simulink model "HANcoder_E407_TTA_Template_group2"  (R2018b)
settings: Solver=FixedStepDiscrete  StartTime=0.0  StopTime=1  FixedStep=0.01  RelTol=1e-3
PreLoadFcn:
  | librarySetup
  | eval([bdroot,'_startup']) %Calling [modelName]_startup.m
values from neighbouring files (symbols this model uses):
  basic_cycle_duration_bc0 = TM_Reset_Board   + COMP_duration    (= 1050)    [HANcoder_E407_TTA_Group2_startup.m]    (also in HANcoder_E407_TTA_Template_startup.m = 212)
  basic_cycle_duration_bc1 = TM_Reset_Var_bc1 + COMP_duration    (= 1070)    [HANcoder_E407_TTA_Group2_startup.m]    (also in HANcoder_E407_TTA_Template_startup.m = 212)
  comm_delay_estimation1 = round(comm_delay_measured1*hardware_granularity/frequency_IRQ)    [HANcoder_E407_TTA_Group2_startup.m]    (also in HANcoder_E407_TTA_Template_startup.m)
  comm_delay_estimation2 = round(comm_delay_measured2*hardware_granularity/frequency_IRQ)    [HANcoder_E407_TTA_Group2_startup.m]    (also in HANcoder_E407_TTA_Template_startup.m)
  COMM_Period = 60    [HANcoder_E407_TTA_Group2_startup.m]    (also in HANcoder_E407_TTA_Template_startup.m = 40)
  COMM_Phase1 = Simulink.Parameter    [HANcoder_E407_TTA_Group2_startup.m]    (also in HANcoder_E407_TTA_Template_startup.m)
  COMM_Phase2 = Simulink.Parameter    [HANcoder_E407_TTA_Group2_startup.m]    (also in HANcoder_E407_TTA_Template_startup.m)
  COMM_Phase_init1 = Simulink.Parameter    [HANcoder_E407_TTA_Group2_startup.m]    (also in HANcoder_E407_TTA_Template_startup.m)
  COMM_Phase_init2 = Simulink.Parameter    [HANcoder_E407_TTA_Group2_startup.m]    (also in HANcoder_E407_TTA_Template_startup.m)
  COMP_duration = 50    [HANcoder_E407_TTA_Group2_startup.m]    (also in HANcoder_E407_TTA_Template_startup.m = 4)
  Controller1_Board = 1    [HANcoder_E407_TTA_Group2_startup.m]    (also in HANcoder_E407_TTA_Template_startup.m)
  Controller2_Board = 2    [HANcoder_E407_TTA_Group2_startup.m]    (also in HANcoder_E407_TTA_Template_startup.m)
  Controller3_Board = 3    [HANcoder_E407_TTA_Group2_startup.m]    (also in HANcoder_E407_TTA_Template_startup.m)
  delta_a_set = Simulink.Parameter    [HANcoder_E407_TTA_Group2_startup.m]
  delta_f_set = Simulink.Parameter    [HANcoder_E407_TTA_Group2_startup.m]
  delta_max = 1    [HANcoder_E407_TTA_Group2_startup.m]
  delta_min = -1    [HANcoder_E407_TTA_Group2_startup.m]
  delta_precision = 6    [HANcoder_E407_TTA_Group2_startup.m]
  frequency_IRQ = 100    [HANcoder_E407_TTA_Group2_startup.m]    (also in HANcoder_E407_TTA_Template_startup.m)
  HANtuneOverride = Simulink.Parameter    [HANcoder_E407_TTA_Group2_startup.m]    (also in HANcoder_E407_TTA_Template_startup.m)
  idle_time_init = basic_cycle_duration_bc0 + basic_cycle_duration_bc1    (= 2120)    [HANcoder_E407_TTA_Group2_startup.m]    (also in HANcoder_E407_TTA_Template_startup.m = 424)
  Input_Gen_Board = 5    [HANcoder_E407_TTA_Group2_startup.m]
  LA_Clock_Gr = 1    [HANcoder_E407_TTA_Group2_startup.m]    (also in HANcoder_E407_TTA_Template_startup.m)
  LA_COMM_dly = 1    [HANcoder_E407_TTA_Group2_startup.m]    (also in HANcoder_E407_TTA_Template_startup.m)
  LA_COMM_Err = 1    [HANcoder_E407_TTA_Group2_startup.m]    (also in HANcoder_E407_TTA_Template_startup.m)
  LA_E_Desync = 1    [HANcoder_E407_TTA_Group2_startup.m]    (also in HANcoder_E407_TTA_Template_startup.m)
  LA_MEX_Flag = 1    [HANcoder_E407_TTA_Group2_startup.m]    (also in HANcoder_E407_TTA_Template_startup.m)
  LA_Task_Act = 1    [HANcoder_E407_TTA_Group2_startup.m]    (also in HANcoder_E407_TTA_Template_startup.m)
  Master_Role = 1    [HANcoder_E407_TTA_Group2_startup.m]    (also in HANcoder_E407_TTA_Template_startup.m)
  matrix_rows = 2    [HANcoder_E407_TTA_Group2_startup.m]    (also in HANcoder_E407_TTA_Template_startup.m)
  max_desync = 30    [HANcoder_E407_TTA_Group2_startup.m]    (also in HANcoder_E407_TTA_Template_startup.m = 15)
  max_num_msgs_CAN1 = 2^Tx_bit_number-1    (= 7)    [HANcoder_E407_TTA_Group2_startup.m]    (also in HANcoder_E407_TTA_Template_startup.m)
  max_num_msgs_CAN2 = max_num_msgs_CAN1    (= 7)    [HANcoder_E407_TTA_Group2_startup.m]    (also in HANcoder_E407_TTA_Template_startup.m)
  min_desync = (-1)*max_desync    (= -30)    [HANcoder_E407_TTA_Group2_startup.m]    (also in HANcoder_E407_TTA_Template_startup.m = -15)
  OutControl1_ID = 23    [HANcoder_E407_TTA_Group2_startup.m]    (also in HANcoder_E407_TTA_Template_startup.m)
  OutControl2_ID = 24    [HANcoder_E407_TTA_Group2_startup.m]    (also in HANcoder_E407_TTA_Template_startup.m)
  OutEmulator_ID = 25    [HANcoder_E407_TTA_Group2_startup.m]    (also in HANcoder_E407_TTA_Template_startup.m)
  script_run = Simulink.Parameter    [HANcoder_E407_TTA_Group2_startup.m]    (also in HANcoder_E407_TTA_Template_startup.m)
  SensorValues_ID = 22    [HANcoder_E407_TTA_Group2_startup.m]    (also in HANcoder_E407_TTA_Template_startup.m)
  SetValues_ID = 21    [HANcoder_E407_TTA_Group2_startup.m]    (also in HANcoder_E407_TTA_Template_startup.m)
  Slave_Role = 3    [HANcoder_E407_TTA_Group2_startup.m]    (also in HANcoder_E407_TTA_Template_startup.m = 2)
  speed_max = 10    [HANcoder_E407_TTA_Group2_startup.m]
  speed_min = -10    [HANcoder_E407_TTA_Group2_startup.m]
  speed_precision = 3    [HANcoder_E407_TTA_Group2_startup.m]
  Sync_ID = 1    [HANcoder_E407_TTA_Group2_startup.m]    (also in HANcoder_E407_TTA_Template_startup.m)
  TM_Check_Sensor_Values = TM_COMM_Sensor_Values + COMM_duration    (= 330)    [HANcoder_E407_TTA_Group2_startup.m]
  TM_Check_Sensor_Values_2 = TM_Check_Sensor_Values + 6    (= 336)    [HANcoder_E407_TTA_Group2_startup.m]
  TM_Check_Set_Values = TM_COMM_Set_Values + COMM_duration    (= 220)    [HANcoder_E407_TTA_Group2_startup.m]
  TM_Check_Set_Values_2 = TM_Check_Set_Values + 6    (= 226)    [HANcoder_E407_TTA_Group2_startup.m]
  TM_Check_Sync = TM_COMM_Sync   + COMM_duration    (= 40)    [HANcoder_E407_TTA_Template_startup.m]
  TM_Check_TOuts = TM_Count_Vote3 + COMP_duration    (= 196)    [HANcoder_E407_TTA_Template_startup.m]
  TM_Check_Vote1 = TM_COMM_Vote1  + COMM_duration    (= 92)    [HANcoder_E407_TTA_Template_startup.m]
  TM_Check_Vote2 = TM_COMM_Vote2  + COMM_duration    (= 140)    [HANcoder_E407_TTA_Template_startup.m]
  TM_Check_Vote3 = TM_COMM_Vote3  + COMM_duration    (= 188)    [HANcoder_E407_TTA_Template_startup.m]
  TM_COMM_Set_Values = TM_bc0_3 + COMP_duration    (= 160)    [HANcoder_E407_TTA_Group2_startup.m]
  TM_COMM_Sync = basic_cycle_start    (= 0)    [HANcoder_E407_TTA_Group2_startup.m]    (also in HANcoder_E407_TTA_Template_startup.m)
  TM_COMM_Vote1 = TM_Vote_Dec    + COMP_duration    (= 52)    [HANcoder_E407_TTA_Template_startup.m]
  TM_COMM_Vote2 = TM_Count_Vote1 + COMP_duration    (= 100)    [HANcoder_E407_TTA_Template_startup.m]
  TM_COMM_Vote3 = TM_Count_Vote2 + COMP_duration    (= 148)    [HANcoder_E407_TTA_Template_startup.m]
  TM_Count_Vote1 = TM_Check_Vote1 + COMP_duration    (= 96)    [HANcoder_E407_TTA_Template_startup.m]
  TM_Count_Vote2 = TM_Check_Vote2 + COMP_duration    (= 144)    [HANcoder_E407_TTA_Template_startup.m]
  TM_Count_Vote3 = TM_Check_Vote3 + COMP_duration    (= 192)    [HANcoder_E407_TTA_Template_startup.m]
  TM_Data_bc0 = TM_COMM_Sync    (= 0)    [HANcoder_E407_TTA_Group2_startup.m]    (also in HANcoder_E407_TTA_Template_startup.m)
  TM_Data_bc1 = TM_Data_bc0(1:4)    [HANcoder_E407_TTA_Group2_startup.m]    (also in HANcoder_E407_TTA_Template_startup.m)
  TM_New_Master = TM_Check_TOuts + COMP_duration    (= 200)    [HANcoder_E407_TTA_Template_startup.m]
  TM_Reset_Board = TM_Reset_Var   + COMP_duration    (= 1000)    [HANcoder_E407_TTA_Group2_startup.m]    (also in HANcoder_E407_TTA_Template_startup.m = 208)
  TM_Reset_Var = TM_bc0_18  + COMP_duration    (= 950)    [HANcoder_E407_TTA_Group2_startup.m]    (also in HANcoder_E407_TTA_Template_startup.m = 204)
  TM_Reset_Var_bc1 = TM_bc1_19 + COMP_duration    (= 1020)    [HANcoder_E407_TTA_Group2_startup.m]    (also in HANcoder_E407_TTA_Template_startup.m = 200)
  TM_Reset_Var_bc1_2 = TM_Reset_Var_bc1 + 6    (= 1026)    [HANcoder_E407_TTA_Group2_startup.m]    (also in HANcoder_E407_TTA_Template_startup.m = 202)
  TM_Type_bc0 = COMM    (= 0)    [HANcoder_E407_TTA_Group2_startup.m]    (also in HANcoder_E407_TTA_Template_startup.m)
  TM_Type_bc1 = TM_Type_bc0(1:4)    [HANcoder_E407_TTA_Group2_startup.m]    (also in HANcoder_E407_TTA_Template_startup.m)
  TM_Update_LT = TM_Check_Sync  + COMP_duration    (= 44)    [HANcoder_E407_TTA_Template_startup.m]
  TM_Update_LT_2 = TM_Update_LT   + 2    (= 46)    [HANcoder_E407_TTA_Template_startup.m]
  TM_Vote_Dec = TM_Update_LT   + COMP_duration    (= 48)    [HANcoder_E407_TTA_Template_startup.m]
  TM_Vote_Dec_2 = TM_Vote_Dec    + 2    (= 50)    [HANcoder_E407_TTA_Template_startup.m]
  v_set = Simulink.Parameter    [HANcoder_E407_TTA_Group2_startup.m]
  Vote1_ID = 11    [HANcoder_E407_TTA_Group2_startup.m]    (also in HANcoder_E407_TTA_Template_startup.m)
  Vote2_ID = 12    [HANcoder_E407_TTA_Group2_startup.m]    (also in HANcoder_E407_TTA_Template_startup.m)
  Vote3_ID = 13    [HANcoder_E407_TTA_Group2_startup.m]    (also in HANcoder_E407_TTA_Template_startup.m)
undefined symbols (not defined in the file or in its folder): A0, A1, A2, A3, A4, CON2, CON4, D10, D12, D13, D8, D9
libraries: hdlsllib x133, HANcoder_STM32_Target x28, simulink x3, simulink_extras x1
(part 1 of 16)
CloseFcn:
  | rtwprivate ssgencode ModelCloseRequest mytest
settings Model: Creator=Jason van Kolfschoten  LastModifiedBy=moham
settings SolverCC: PositivePriorityOrder=on
settings DataIOCC: LimitDataPoints=on  SaveFormat=Array  SignalLoggingSaveFormat=ModelDataLogs  SaveOutput=off  SignalLogging=off  DSMLogging=off  SaveTime=off
settings OptimizationCC: BlockReduction=off  DefaultParameterBehavior=Inlined  DefaultUnderspecifiedDataType=single  InlineInvariantSignals=on  ExpressionDepthLimit=2147483647  StateBitsets=on  DataBitsets=on  ZeroExternalMemoryAtStartup=off  ZeroInternalMemoryAtStartup=off  InitFltsAndDblsToZero=on  NoFixptDivByZeroProtection=on  EfficientFloat2IntCast=on  LifeSpan=inf
settings DebuggingCC: SaveWithDisabledLinksMsg=none  SaveWithParameterizedLinksMsg=none  CheckSSInitialOutputMsg=off  UnderspecifiedInitializationDetection=Classic  MergeDetectMultiDrivingBlocksExec=none  SignalResolutionControl=TryResolveAll  SolverPrmCheckMsg=warning  InheritedTsInSrcMsg=none  MultiTaskDSMMsg=warning  MultiTaskCondExecSysMsg=none  ParameterPrecisionLossMsg=none  FcnCallInpInsideContextMsg=warning  BusObjectLabelMismatch=none  StateNameClashWarn=warning  SFUnexpectedBacktrackingDiag=warning  SFNoUnconditionalDefaultTransitionDiag=warning  SFExecutionAtInitializationDiag=none
settings HardwareCC: ProdBitPerPointer=32  ProdBitPerSizeT=32  ProdBitPerPtrDiffT=32  ProdLargestAtomicInteger=Long  ProdLargestAtomicFloat=Double  ProdWordSize=32  ProdHWDeviceType=ARM Compatible->ARM Cortex  TargetEndianess=LittleEndian  TargetHWDeviceType=Infineon->TriCore
settings ModelReferenceCC: PropagateSignalLabelsOutOfModel=off
settings SFSimCC: SimUseLocalCustomCode=off  MATLABDynamicMemAlloc=off
settings RTWCC: SystemTargetFile=ert.tlc  MakeCommand=make_rtw SHELL= HANcoder_PORTABLE=1 HANcoder_BOOTLOADER=1  TemplateMakefile=STM32_E407_gcc.tmf  Description=Real-Time Workshop Embedded Coder (no auto configuration)  RTWUseLocalCustomCode=off
settings CodeAppCC: ForceParamTrailComments=on  IgnoreCustomStorageClasses=off  SimulinkDataObjDesc=on  CustomSymbolStrGlobalVar=rt$N$M  CustomSymbolStrType=$N$M  CustomSymbolStrFcn=$N$M$F  CustomSymbolStrMacro=$N$M  InsertBlockDesc=on  StateflowObjectComments=on  InternalIdentifier=Classic
settings ERTTargetCC: TargetFcnLib=ansi_tfl_tmw.mat  MultiwordLength=2048  IncludeMdlTerminateFcn=off  SuppressErrorStatus=on  SupportNonFinite=off  SupportVariableSizeSignals=on  GenerateASAP2=on  InlinedParameterPlacement=NonHierarchical  ERTCustomFileTemplate=example_file_process.tlc  ConvertIfToSwitch=off  SuppressUnreachableDefaultCases=off
settings ConfigComp: CovMetricSettings=dw  CovHtmlReporting=on  CovSaveCumulativeToWorkspaceVar=on  CovSaveSingleToWorkspaceVar=on  CovExternalEMLEnable=off  CovSFcnEnable=off  DVMaxProcessTime=600  DVDisplayUnsatisfiableObjectives=on  DVAutomaticStubbing=off  DVModelCoverageObjectives=MCDC  DVMaxTestCaseSteps=500  DVTestSuiteOptimization=CombinedObjectives  DVDetectActiveLogic=on  DVSaveHarnessModel=on

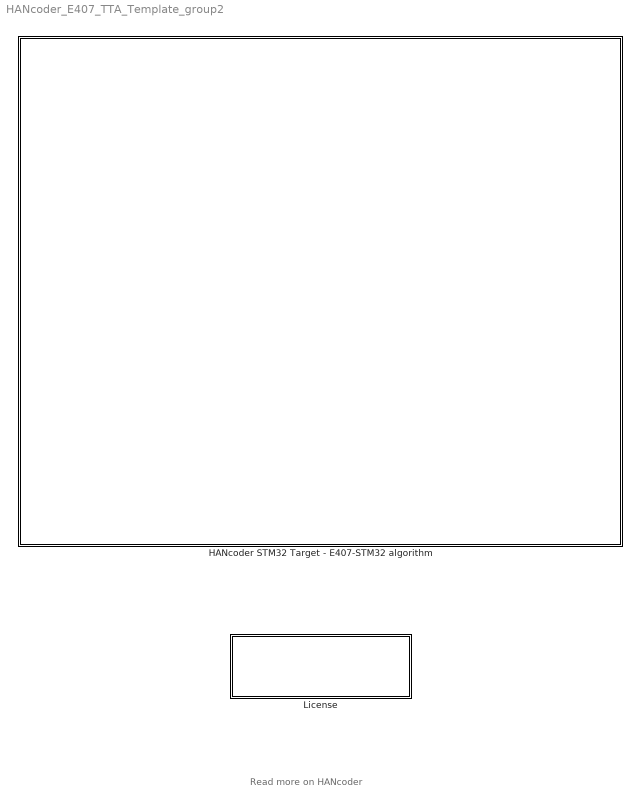
== system HANcoder_E407_TTA_Template_group2 ==
  note: Read more on HANcoder
  HANcoder STM32 Target - E407-STM32 algorithm : Subsystem  mask(TopLevelSubsystem){}
      settings: CopyFcn=HANcoderChecks('Copy');  NameChangeFcn=HANcoderChecks('NameChangeE407');  MoveFcn=HANcoderChecks('MoveE407');
      mask Display: image(imread('STM32_E407_HAN.jpg'))
  License : Subsystem  mask(License){}
      settings: NameChangeFcn=HANcoderChecks('NameChangeLicenseBlock');  OpenFcn=winopen('License.pdf')  MoveFcn=HANcoderChecks('MoveLicenseBlock');
      mask Display: disp(['End-User License Agreement\n','please read before use']);

== system HANcoder_E407_TTA_Template_group2/HANcoder STM32 Target - E407-STM32 algorithm ==
  note: Template model
  Algorithm : Subsystem
  Base Sample Time config : HANcoder_STM32_Target/STM32-E407/System Config/Base Sample Time config  Tag=HANcoder_TARGET_STM32_E407  Description=HANcoder Target STM32-E407 blockset version 1.0  baseSampleTime=10  extraStack=100
      settings: SourceProductName=HANcoder STM32 Target
  Build settings : HANcoder_STM32_Target/STM32-E407/System Config/Build settings  Tag=HANcoder_TARGET_STM32_E407  AutoASAP2add=on  AutoFlash=USB
      settings: SourceProductName=HANcoder STM32 Target
  CAN config : HANcoder_STM32_Target/STM32-E407/System Config/CAN config  Tag=HANcoder_TARGET_STM32_E407  txBufSize=64  evBufSize=8  canBus1=on  baudRate1=1000  rxMask1=hex2dec('00000000')  rxCode1=hex2dec('00000000')  rxMode1=Receive only 11-bit message identifiers  canBus2=on  baudRate2=1000  rxMask2=hex2dec('00000000')  rxCode2=hex2dec('00000000')  rxMode2=Receive only 11-bit message identifiers
      settings: SourceProductName=HANcoder STM32 Target
  Custom ID config : HANcoder_STM32_Target/STM32-E407/System Config/Custom ID config  Tag=HANcoder_TARGET_STM32_E407  softID=softwareID  softNUM=1
      settings: SourceProductName=HANcoder STM32 Target
  Inputs : Subsystem
  Operation Mode : Subsystem
  Outputs : Subsystem
  System information : Subsystem
  TTA CAN System : Subsystem
  XCP on USB config : HANcoder_STM32_Target/STM32-E407/System Config/XCP on USB config  Tag=HANcoder_TARGET_STM32_E407
      settings: SourceProductName=HANcoder STM32 Target
  wires:
  Algorithm/1(LED) -> Outputs/1(LED)
  Inputs/1(Button) -> Operation Mode/1(Button_State), Algorithm/1(Button)
  Operation Mode/1(Clock_State) -> TTA CAN System/1(Clock_State)

== system HANcoder_E407_TTA_Template_group2/License ==

== system HANcoder_E407_TTA_Template_group2/HANcoder STM32 Target - E407-STM32 algorithm/Algorithm ==
  note: The button or the HANtuneOverride parameter
      | switches between the two frequencies.
  note: Here the algorithm can be placed. No hardware dependent blocks should be used here.
  note: Switch LED frequency when button is pressed
  Button : Inport
  10Hz Counter Limiter : simulink/Sources/Counter Limited  uplimit=1  tsamp=0.1
  5Hz Counter Limited : simulink/Sources/Counter Limited  uplimit=1  tsamp=0.2
  Constant : Constant  Value=HANtuneOverride  OutDataTypeStr=boolean
  Data Type Conversion : DataTypeConversion  OutDataTypeStr=boolean
  Logical Operator : Logic  Operator=OR  AllPortsSameDT=off  OutDataTypeStr=boolean
  Switch : Switch  Criteria=u2 > Threshold
  LED : Outport
  wires:
  Data Type Conversion/1 -> LED/1  "LedValue"
  5Hz Counter Limited/1 -> Switch/3
  Switch/1 -> Data Type Conversion/1
  Button/1 -> Logical Operator/2
  Logical Operator/1 -> Switch/2
  Constant/1 -> Logical Operator/1
  10Hz Counter Limiter/1 -> Switch/1

== system HANcoder_E407_TTA_Template_group2/HANcoder STM32 Target - E407-STM32 algorithm/Inputs ==
  note: The inputs and outputs are kept in a separate subsystem, this way the algorithm can easily be transferred to different hardware
  Digital Input : HANcoder_STM32_Target/STM32-E407/Digital Inputs/Digital Input  Tag=HANcoder_TARGET_STM32_E407  pinID=WKUP button  config=Pulldown  tsamp=-1
      settings: SourceProductName=HANcoder STM32 Target
  Button : Outport
  wires:
  Digital Input/1 -> Button/1

== system HANcoder_E407_TTA_Template_group2/HANcoder STM32 Target - E407-STM32 algorithm/Operation Mode ==
  note: Operation Mode
      | There are two modes of operation:
      | ( 0 ) Idle (Clock Off)
      | ( 1 ) Counting (Clock On)
      | In order to switch from one to the other the wake-up button
      | must be pressed once. In this subsystem, with every negative
      | edge of the Button State, the Operation Mode will change from
      | one to the other.
  Button_State : Inport
  Constant : Constant  OutDataTypeStr=boolean
  Flip Flop T : Subsystem
  Clock_State : Outport
  wires:
  Constant/1 -> Flip Flop T/1(T)
  Button_State/1 -> Flip Flop T/2(Clk)
  Flip Flop T/1(Q) -> Clock_State/1

== system HANcoder_E407_TTA_Template_group2/HANcoder STM32 Target - E407-STM32 algorithm/Outputs ==
  note: The inputs and outputs are kept in a separate subsystem, this way the algorithm can easily be transferred to different hardware
  LED : Inport
  Digital Output : HANcoder_STM32_Target/STM32-E407/Digital Outputs/Digital Output  Tag=HANcoder_TARGET_STM32_E407  pinID=LED  config=Push pull  tsamp=-1
      settings: SourceProductName=HANcoder STM32 Target
  wires:
  LED/1 -> Digital Output/1

== system HANcoder_E407_TTA_Template_group2/HANcoder STM32 Target - E407-STM32 algorithm/System information ==
  note: These blocks check the free memory: stack and heap and the CPU load,
      | this way you can see whether your software demands too much of the microcontroller
  Get CPU load : HANcoder_STM32_Target/STM32-E407/System Management/Get CPU load  Tag=HANcoder_TARGET_STM32_E407  mode=Current CPU load  tsamp=-1
      settings: SourceProductName=HANcoder STM32 Target
  Get free Heap : HANcoder_STM32_Target/STM32-E407/System Management/Get free Heap  Tag=HANcoder_TARGET_STM32_E407  tsamp=-1
      settings: SourceProductName=HANcoder STM32 Target
  Get free Stack : HANcoder_STM32_Target/STM32-E407/System Management/Get free Stack  Tag=HANcoder_TARGET_STM32_E407  taskIdx=Application Control Task  tsamp=-1
      settings: SourceProductName=HANcoder STM32 Target
  Terminator : Terminator
  Terminator1 : Terminator
  Terminator2 : Terminator
  wires:
  Get CPU load/1 -> Terminator1/1  "SI_CPUload"
  Get free Stack/1 -> Terminator/1  "SI_FreeStack"
  Get free Heap/1 -> Terminator2/1  "SI_FreeHeap"

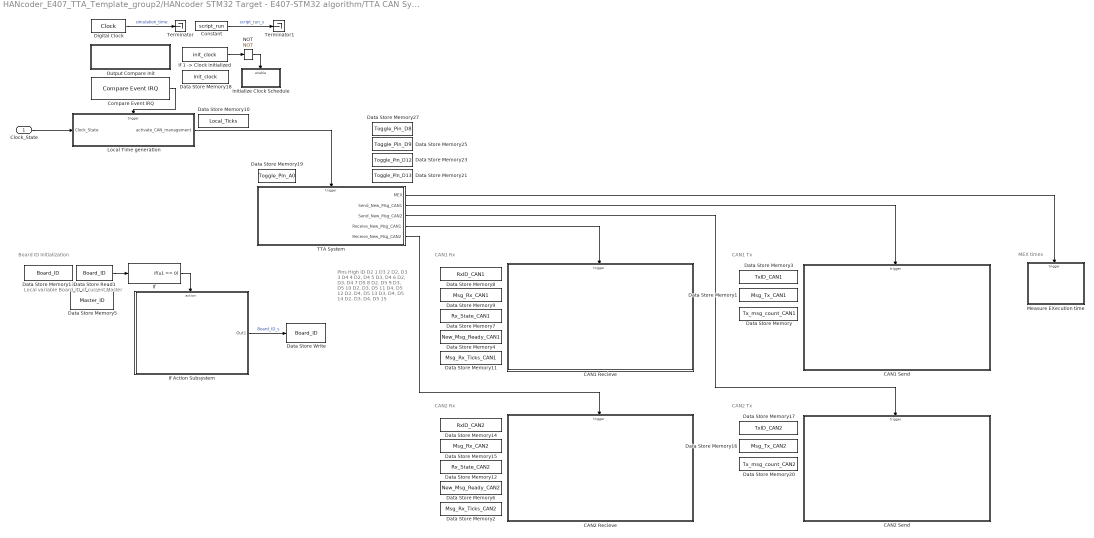
== system HANcoder_E407_TTA_Template_group2/HANcoder STM32 Target - E407-STM32 algorithm/TTA CAN System ==
  note: MEX times
  note: Pins High      		ID
      | D2                 		1
      | D3				2
      | D2, D3			3
      | D4				4
      | D2, D4			5
      | D3, D4			6
      | D2, D3, D4		7
      | D5				8
      | D2, D5			9
      | D3, D5			10
      | D2, D3, D5		11
      | D4, D5			12
      | D2, D4, D5		13
      | D3, D4, D5		14
      | D2, D3, D4, D5	15
  note: Board ID Initialization
  note: Local variable
      | Board_ID of
      | current Master
  note: CAN1 Tx
  note: CAN1 Rx
  note: CAN2 Rx
  note: CAN2 Tx
  Clock_State : Inport
  CAN1 Recieve : Subsystem
  CAN1 Send : Subsystem
  CAN2 Recieve : Subsystem
  CAN2 Send : Subsystem
  Compare Event IRQ : HANcoder_STM32_Target/STM32-E407/Timer Outputs/Compare Event IRQ  Tag=HANcoder_TARGET_STM32_E407  Priority=20  pin=TIM4 - CON PD - 15 - 5V Tolerant
      settings: SourceProductName=HANcoder STM32 Target
  Constant : Constant  Value=script_run
  Data Store Memory : DataStoreMemory  DataStoreName=Tx_msg_count_CAN1  ReadBeforeWriteMsg=warning  WriteAfterWriteMsg=warning  WriteAfterReadMsg=warning  InitialValue=1  ShowAdditionalParam=off
  Data Store Memory1 : DataStoreMemory  Priority=25  DataStoreName=Msg_Tx_CAN1  ReadBeforeWriteMsg=warning  WriteAfterWriteMsg=warning  WriteAfterReadMsg=warning  ShowAdditionalParam=off  OutDataTypeStr=Bus: msg_buffer_type
  Data Store Memory10 : DataStoreMemory  Priority=7  DataStoreName=Local_Ticks  ReadBeforeWriteMsg=warning  WriteAfterWriteMsg=warning  WriteAfterReadMsg=warning  ShowAdditionalParam=off  OutDataTypeStr=uint16
  Data Store Memory11 : DataStoreMemory  Priority=25  DataStoreName=Msg_Rx_Ticks_CAN1  ReadBeforeWriteMsg=warning  WriteAfterWriteMsg=warning  WriteAfterReadMsg=warning  ShowAdditionalParam=off  OutDataTypeStr=uint16
  Data Store Memory12 : DataStoreMemory  Priority=25  DataStoreName=Rx_State_CAN2  ReadBeforeWriteMsg=warning  WriteAfterWriteMsg=warning  WriteAfterReadMsg=warning  ShowAdditionalParam=off  OutDataTypeStr=uint8
  Data Store Memory13 : DataStoreMemory  Priority=10  DataStoreName=Board_ID  ReadBeforeWriteMsg=warning  WriteAfterWriteMsg=warning  WriteAfterReadMsg=warning  ShowAdditionalParam=off
  Data Store Memory14 : DataStoreMemory  Priority=25  DataStoreName=RxID_CAN2  ReadBeforeWriteMsg=warning  WriteAfterWriteMsg=warning  WriteAfterReadMsg=warning  InitialValue=Sync_ID  ShowAdditionalParam=off  OutDataTypeStr=uint32
  Data Store Memory15 : DataStoreMemory  Priority=25  DataStoreName=Msg_Rx_CAN2  ReadBeforeWriteMsg=warning  WriteAfterWriteMsg=warning  WriteAfterReadMsg=warning  ShowAdditionalParam=off  OutDataTypeStr=Bus: msg_buffer_type
  Data Store Memory16 : DataStoreMemory  Priority=25  DataStoreName=Msg_Tx_CAN2  ReadBeforeWriteMsg=warning  WriteAfterWriteMsg=warning  WriteAfterReadMsg=warning  ShowAdditionalParam=off  OutDataTypeStr=Bus: msg_buffer_type
  Data Store Memory17 : DataStoreMemory  Priority=25  DataStoreName=TxID_CAN2  ReadBeforeWriteMsg=warning  WriteAfterWriteMsg=warning  WriteAfterReadMsg=warning  ShowAdditionalParam=off  OutDataTypeStr=uint32
  Data Store Memory18 : DataStoreMemory  Priority=1  DataStoreName=init_clock  ReadBeforeWriteMsg=warning  WriteAfterWriteMsg=warning  WriteAfterReadMsg=warning  ShowAdditionalParam=off
  Data Store Memory19 : DataStoreMemory  Priority=9  DataStoreName=Toggle_Pin_A0  ReadBeforeWriteMsg=warning  WriteAfterWriteMsg=warning  WriteAfterReadMsg=warning  ShowAdditionalParam=off
  Data Store Memory2 : DataStoreMemory  Priority=25  DataStoreName=Msg_Rx_Ticks_CAN2  ReadBeforeWriteMsg=warning  WriteAfterWriteMsg=warning  WriteAfterReadMsg=warning  ShowAdditionalParam=off  OutDataTypeStr=uint16
  Data Store Memory20 : DataStoreMemory  DataStoreName=Tx_msg_count_CAN2  ReadBeforeWriteMsg=warning  WriteAfterWriteMsg=warning  WriteAfterReadMsg=warning  InitialValue=1  ShowAdditionalParam=off
  Data Store Memory21 : DataStoreMemory  Priority=9  DataStoreName=Toggle_Pin_D13  ReadBeforeWriteMsg=warning  WriteAfterWriteMsg=warning  WriteAfterReadMsg=warning  ShowAdditionalParam=off
  Data Store Memory23 : DataStoreMemory  Priority=9  DataStoreName=Toggle_Pin_D12  ReadBeforeWriteMsg=warning  WriteAfterWriteMsg=warning  WriteAfterReadMsg=warning  ShowAdditionalParam=off
  Data Store Memory25 : DataStoreMemory  Priority=9  DataStoreName=Toggle_Pin_D9  ReadBeforeWriteMsg=warning  WriteAfterWriteMsg=warning  WriteAfterReadMsg=warning  ShowAdditionalParam=off
  Data Store Memory27 : DataStoreMemory  Priority=9  DataStoreName=Toggle_Pin_D8  ReadBeforeWriteMsg=warning  WriteAfterWriteMsg=warning  WriteAfterReadMsg=warning  ShowAdditionalParam=off
  Data Store Memory3 : DataStoreMemory  Priority=25  DataStoreName=TxID_CAN1  ReadBeforeWriteMsg=warning  WriteAfterWriteMsg=warning  WriteAfterReadMsg=warning  ShowAdditionalParam=off  OutDataTypeStr=uint32
  Data Store Memory4 : DataStoreMemory  Priority=25  DataStoreName=New_Msg_Ready_CAN1  ReadBeforeWriteMsg=warning  WriteAfterWriteMsg=warning  WriteAfterReadMsg=warning  ShowAdditionalParam=off  OutDataTypeStr=boolean
  Data Store Memory5 : DataStoreMemory  Priority=10  DataStoreName=Master_ID  ReadBeforeWriteMsg=warning  WriteAfterWriteMsg=warning  WriteAfterReadMsg=warning  InitialValue=1  ShowAdditionalParam=off
  Data Store Memory6 : DataStoreMemory  Priority=25  DataStoreName=New_Msg_Ready_CAN2  ReadBeforeWriteMsg=warning  WriteAfterWriteMsg=warning  WriteAfterReadMsg=warning  ShowAdditionalParam=off  OutDataTypeStr=boolean
  Data Store Memory7 : DataStoreMemory  Priority=25  DataStoreName=Rx_State_CAN1  ReadBeforeWriteMsg=warning  WriteAfterWriteMsg=warning  WriteAfterReadMsg=warning  ShowAdditionalParam=off  OutDataTypeStr=uint8
  Data Store Memory8 : DataStoreMemory  Priority=25  DataStoreName=RxID_CAN1  ReadBeforeWriteMsg=warning  WriteAfterWriteMsg=warning  WriteAfterReadMsg=warning  InitialValue=Sync_ID  ShowAdditionalParam=off  OutDataTypeStr=uint32
  Data Store Memory9 : DataStoreMemory  Priority=25  DataStoreName=Msg_Rx_CAN1  ReadBeforeWriteMsg=warning  WriteAfterWriteMsg=warning  WriteAfterReadMsg=warning  ShowAdditionalParam=off  OutDataTypeStr=Bus: msg_buffer_type
  Data Store Read1 : DataStoreRead  Priority=10  DataStoreName=Board_ID
  Data Store Write : DataStoreWrite  Priority=13  DataStoreName=Board_ID
  Digital Clock : DigitalClock  Priority=1  SampleTime=0.01
  If : If  Priority=11  IfExpression=u1 == 0  ShowElse=off
  "If 1 -> Clock initialized " : DataStoreRead  Priority=2  DataStoreName=init_clock
  If Action Subsystem : Subsystem  Priority=12  TreatAsAtomicUnit=on
  Initialize Clock Schedule : Subsystem  Priority=4  TreatAsAtomicUnit=on
  Local Time generation : Subsystem  TreatAsAtomicUnit=on
  Measure EXecution time : Subsystem  TreatAsAtomicUnit=on
  NOT : Logic  Priority=3  Operator=NOT  IconShape=distinctive  AllPortsSameDT=off  OutDataTypeStr=boolean
  Output Compare Init : Subsystem  Tag=HANcoder_TARGET_STM32_E407  AncestorBlock=HANcoder_STM32_Target/STM32-E407/Timer Outputs/Output Compare Init  mask(Output Compare Init){moduleID=TIM4 - CON PD - 15 & 16 &n/a & n/a, frequency=1000000, enableIRQoutput=off}
      mask prompts: moduleID "Timer module"; frequency "Frequency (free running counter) [Hz]"; enableIRQoutput "Enable IRQ output"
      mask help:
      | Function
      | ========
      | Initializes the timer module to allow output compare functionality on the
      | module's channels.
      |
      | Parameters
      | ==========
      | Timer Module:
      |   Selects the timer module.
      |
      | Frequency:
      |   Frequency at which the 16-bit free running counter counts.
      |
      | Enable IRQ output
      |   Controls whether or not the IRQ output is available.
      |
      | Outport
      | =======
      | IRQ
      |   Allows connection of a function call subsystem for the free running
      |   counter overflow event.
      mask init:
      | moduleIDInfoStr = sfcn_timeout_init_mcb(2, moduleID, frequency, enableIRQoutput);
      settings: CopyFcn=sfcn_timeout_init_chk();  MoveFcn=drawLogos
      mask Help: web('sfcn_timeout_init.html');
      mask TypeOptions moduleID: TIM1 - CON PE - 12 & 14 & 16 & 17 | TIM2 - CON4 - D13 & n/a & n/a & n/a | TIM3 - CON4 - D12 & D11 & n/a & n/a | TIM4 - CON PD - 15 & 16 &n/a & n/a | TIM8 - UEXT - 3 & 4 & n/a & n/a | TIM9 - CON3 - D4 & D5 or PE - 8 & 9 | TIM10 - CON2 - A1 or CON PF - 9 | TIM11 - CON2 - A2 or CON PF - 10 | TIM13 - CON2 - A3 or CON PF - 11 | TIM14 - CON2 - A4 or CON PF - 12
      mask Callback moduleID: sfcn_timeout_init_chk();
      mask Display: fprintf('Output Compare Init\n%s', moduleIDInfoStr);patch([135 141 141],[8 14 2],[1 0 0]);patch([143 143 149],[14 2 8],[0 0 0.35]);
  TTA System : Subsystem
  Terminator : Terminator
  Terminator1 : Terminator
  wires:
  Digital Clock/1 -> Terminator/1  "simulation_time"
  If/1 -> If Action Subsystem/Action
  Data Store Read1/1 -> If/1
  If Action Subsystem/1(Out1) -> Data Store Write/1  "Board_ID_s"
  TTA System/2(Send_New_Msg_CAN1) -> CAN1 Send/Trigger
  TTA System/4(Receive_New_Msg_CAN1) -> CAN1 Recieve/Trigger
  TTA System/5(Receive_New_Msg_CAN2) -> CAN2 Recieve/Trigger
  TTA System/3(Send_New_Msg_CAN2) -> CAN2 Send/Trigger
  TTA System/1(MEX) -> Measure EXecution time/Trigger
  Local Time generation/1(activate_CAN_management) -> TTA System/Trigger
  NOT/1 -> Initialize Clock Schedule/Enable
  Compare Event IRQ/1 -> Local Time generation/Trigger
  "If 1 -> Clock initialized "/1 -> NOT/1
  Clock_State/1 -> Local Time generation/1(Clock_State)
  Constant/1 -> Terminator1/1  "script_run_s"

== system HANcoder_E407_TTA_Template_group2/HANcoder STM32 Target - E407-STM32 algorithm/Operation Mode/Flip Flop T ==
  T : Inport  OutDataTypeStr=boolean
  Clk : Inport  Port=2  OutDataTypeStr=boolean
  J-K Flip-Flop : simulink_extras/Flip Flops/J-K Flip-Flop  initial_condition=0
      settings: SourceProductName=Simulink
  Terminator : Terminator
  Q : Outport  OutDataTypeStr=boolean
  wires:
  J-K Flip-Flop/2 -> Terminator/1
  T/1 -> J-K Flip-Flop/3, J-K Flip-Flop/1
  J-K Flip-Flop/1 -> Q/1
  Clk/1 -> J-K Flip-Flop/2

== system HANcoder_E407_TTA_Template_group2/HANcoder STM32 Target - E407-STM32 algorithm/TTA CAN System/CAN1 Recieve ==
  note: Function call counter
  Trigger : TriggerPort  TriggerType=function-call  VariantControl=Variant  PortDimensions=1
  AND2 : Logic  IconShape=distinctive  AllPortsSameDT=off  OutDataTypeStr=boolean
  AND3 : Logic  IconShape=distinctive  AllPortsSameDT=off  OutDataTypeStr=boolean
  Buffer ready : Subsystem  TreatAsAtomicUnit=on
  Constant : Constant  Value=0
  Constant3 : Constant  OutDataTypeStr=uint32
  Constant4 : Constant
  Constant5 : Constant  Value=2
  Constant6 : Constant  Value=0
  Constant7 : Constant
  Data Store Memory1 : DataStoreMemory  DataStoreName=fcn_call_counter  ReadBeforeWriteMsg=warning  WriteAfterWriteMsg=warning  WriteAfterReadMsg=warning  ShowAdditionalParam=off  OutDataTypeStr=uint32
  Data Store Read : DataStoreRead  DataStoreName=RxID_CAN1
  Data Store Read1 : DataStoreRead  DataStoreName=fcn_call_counter
  Data Store Read10 : DataStoreRead  DataStoreName=Rx_State_CAN1
  Data Store Read4 : DataStoreRead  DataStoreName=Rx_State_CAN1
  Data Store Read9 : DataStoreRead  DataStoreName=Rx_State_CAN1
  Data Store Write : DataStoreWrite  DataStoreName=fcn_call_counter
  Equal{3,5..7} (4 alike) : RelationalOperator  Operator===  OutDataTypeStr=boolean  RndMeth=Simplest
  Equal4 : RelationalOperator  OutDataTypeStr=boolean  RndMeth=Simplest
  Prepare buffer : Subsystem  TreatAsAtomicUnit=on
  RxID_CAN : Subsystem
  Sum1 : Sum
  Update message buffers : Subsystem
  wires:
  AND3/1 -> Update message buffers/Enable
  Data Store Read/1 -> RxID_CAN/1(RxID)  "RxID_CAN1_s"
  RxID_CAN/2(message) -> Update message buffers/1(message)
  Constant7/1 -> Equal6/2
  Constant6/1 -> Equal5/2
  RxID_CAN/1(CAN_new) -> Equal4/1, Equal3/2
  Constant5/1 -> Equal7/2
  Equal5/1 -> Prepare buffer/Enable
  Data Store Read9/1 -> Equal7/1
  Equal4/1 -> AND3/2
  Equal6/1 -> AND2/1
  Equal3/1 -> AND2/2
  AND2/1 -> Buffer ready/Enable
  Equal7/1 -> AND3/1
  Data Store Read10/1 -> Equal6/1
  Constant/1 -> Equal3/1
  Data Store Read4/1 -> Equal5/1
  Data Store Read1/1 -> Sum1/2
  Constant3/1 -> Sum1/1
  Sum1/1 -> Data Store Write/1  "RxCAN1_counter_s"
  Constant4/1 -> Equal4/2

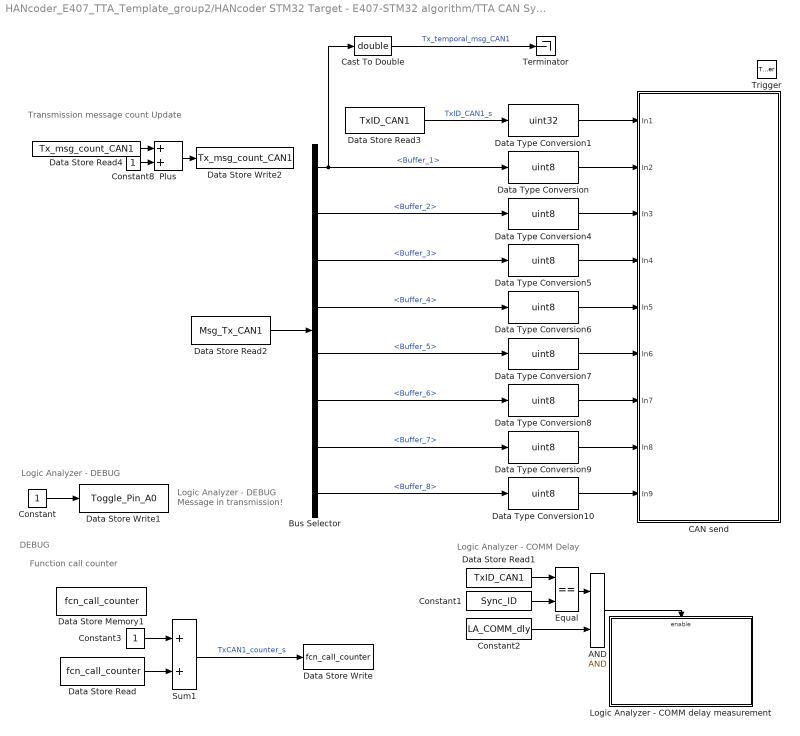
== system HANcoder_E407_TTA_Template_group2/HANcoder STM32 Target - E407-STM32 algorithm/TTA CAN System/CAN1 Send ==
  note: Logic Analyzer - COMM Delay
  note: Logic Analyzer - DEBUG
  note: DEBUG
  note: Function call counter
  note: Logic Analyzer - DEBUG
      | Message in transmission!
  note: Transmission message count
      | Update
  Trigger : TriggerPort  TriggerType=function-call  VariantControl=Variant  PortDimensions=1
  AND : Logic  IconShape=distinctive  AllPortsSameDT=off  OutDataTypeStr=boolean
  Bus Selector : BusSelector  OutputSignals=Buffer_1,Buffer_2,Buffer_3,Buffer_4,Buffer_5,Buffer_6,Buffer_7,Buffer_8
  CAN send : Subsystem  Tag=HANcoder_TARGET_STM32_E407  AncestorBlock=HANcoder_STM32_Target/STM32-E407/CAN/CAN/CAN send  mask(CAN send){canBus=CAN 1, frameType=Standard (11 bit), inputNumber=8, dataType=uint8, byteOrder=off, tsamp=-1}
      mask prompts: canBus "CAN channel"; frameType "Identifier type"; inputNumber "Input ports"; dataType "Input datatype"; byteOrder "Byte order: Checked = MSB first, unchecked = LSB first."; tsamp "Sample time"
      mask help:
      | Function
      | ==========
      | Send a message on the CAN channel.
      |
      | Parameters
      | ==========
      | CAN channel:           The CAN channel to send the message on.
      | Identifier type:         normal or extended ID's
      | Input ports:              The amount of input ports
      | Input datatype:        The datatype of the input ports
      | Byte order:               Select MSB or LSB first
      | Sample time:            -1 or divisible by base sample time [seconds]
      |
      | Input
      | ==========
      | Port 1:                   CAN ID(uint32) in hexadecimal ie: hex2dec('0a')
      | Port 2..9                CAN message data
      mask init:
      | sfcn_can_send_mcb(canBus, frameType, inputNumber, dataType, byteOrder)
      settings: MoveFcn=drawLogos
      mask Help: web('sfcn_can_send.html');
      mask TypeOptions canBus: CAN 1 | CAN 2
      mask TypeOptions frameType: Standard (11 bit) | Extended (29 bit)
      mask TypeOptions dataType: int8 | uint8 | int16 | uint16 | int32 | uint32 | boolean
      mask Display:
      | fprintf('Send on\nCAN %x', canBus);
      | port_label('input', 1, 'ID');patch([135 141 141],[8 14 2],[1 0 0]);patch([143 143 149],[14 2 8],[0 0 0.35]);
  Cast To Double : DataTypeConversion  OutDataTypeStr=double
  Constant : Constant  OutDataTypeStr=boolean
  Constant1 : Constant  Value=Sync_ID
  Constant2 : Constant  Value=LA_COMM_dly
  Constant3 : Constant  OutDataTypeStr=uint32
  Constant8 : Constant  Priority=2
  Data Store Memory1 : DataStoreMemory  DataStoreName=fcn_call_counter  ReadBeforeWriteMsg=warning  WriteAfterWriteMsg=warning  WriteAfterReadMsg=warning  ShowAdditionalParam=off  OutDataTypeStr=uint32
  Data Store Read : DataStoreRead  DataStoreName=fcn_call_counter
  Data Store Read1 : DataStoreRead  DataStoreName=TxID_CAN1
  Data Store Read2 : DataStoreRead  DataStoreName=Msg_Tx_CAN1
  Data Store Read3 : DataStoreRead  DataStoreName=TxID_CAN1
  Data Store Read4 : DataStoreRead  Priority=1  DataStoreName=Tx_msg_count_CAN1
  Data Store Write : DataStoreWrite  DataStoreName=fcn_call_counter
  Data Store Write1 : DataStoreWrite  DataStoreName=Toggle_Pin_A0
  Data Store Write2 : DataStoreWrite  Priority=4  DataStoreName=Tx_msg_count_CAN1
  Data Type Conversion{,4..10} (8 alike) : DataTypeConversion  OutDataTypeStr=uint8
  Data Type Conversion1 : DataTypeConversion  OutDataTypeStr=uint32
  Equal : RelationalOperator  Operator===  OutDataTypeStr=boolean  RndMeth=Simplest
  Logic Analyzer - COMM delay measurement : Subsystem  TreatAsAtomicUnit=on
  Plus : Sum  Priority=3
  Sum1 : Sum
  Terminator : Terminator
  wires:
  Data Type Conversion10/1 -> CAN send/9(In9)
  Data Type Conversion/1 -> CAN send/2(In2)
  Data Type Conversion1/1 -> CAN send/1(In1)
  Data Type Conversion9/1 -> CAN send/8(In8)
  Data Type Conversion8/1 -> CAN send/7(In7)
  Data Type Conversion5/1 -> CAN send/4(In4)
  Data Type Conversion4/1 -> CAN send/3(In3)
  Data Type Conversion6/1 -> CAN send/5(In5)
  Data Type Conversion7/1 -> CAN send/6(In6)
  Constant3/1 -> Sum1/1
  Data Store Read/1 -> Sum1/2
  Sum1/1 -> Data Store Write/1  "TxCAN1_counter_s"
  Constant/1 -> Data Store Write1/1
  Data Store Read2/1 -> Bus Selector/1
  Bus Selector/2 -> Data Type Conversion4/1  "<Buffer_2>"
  Bus Selector/3 -> Data Type Conversion5/1  "<Buffer_3>"
  Bus Selector/4 -> Data Type Conversion6/1  "<Buffer_4>"
  Bus Selector/5 -> Data Type Conversion7/1  "<Buffer_5>"
  Bus Selector/6 -> Data Type Conversion8/1  "<Buffer_6>"
  Bus Selector/7 -> Data Type Conversion9/1  "<Buffer_7>"
  Bus Selector/8 -> Data Type Conversion10/1  "<Buffer_8>"
  Data Store Read3/1 -> Data Type Conversion1/1  "TxID_CAN1_s"
  Constant8/1 -> Plus/2
  Plus/1 -> Data Store Write2/1
  Data Store Read4/1 -> Plus/1
  Cast To Double/1 -> Terminator/1  "Tx_temporal_msg_CAN1"
  Bus Selector/1 -> Cast To Double/1, Data Type Conversion/1  "<Buffer_1>"
  Data Store Read1/1 -> Equal/1
  Constant1/1 -> Equal/2
  Constant2/1 -> AND/2
  AND/1 -> Logic Analyzer - COMM delay measurement/Enable
  Equal/1 -> AND/1

== system HANcoder_E407_TTA_Template_group2/HANcoder STM32 Target - E407-STM32 algorithm/TTA CAN System/CAN2 Recieve ==
  note: Function call counter
  Trigger : TriggerPort  TriggerType=function-call  VariantControl=Variant  PortDimensions=1
  AND2 : Logic  IconShape=distinctive  AllPortsSameDT=off  OutDataTypeStr=boolean
  AND3 : Logic  IconShape=distinctive  AllPortsSameDT=off  OutDataTypeStr=boolean
  Buffer ready : Subsystem  TreatAsAtomicUnit=on
  Constant : Constant  Value=0
  Constant3 : Constant  OutDataTypeStr=uint32
  Constant4 : Constant
  Constant5 : Constant  Value=2
  Constant6 : Constant  Value=0
  Constant7 : Constant
  Data Store Memory1 : DataStoreMemory  DataStoreName=fcn_call_counter  ReadBeforeWriteMsg=warning  WriteAfterWriteMsg=warning  WriteAfterReadMsg=warning  ShowAdditionalParam=off  OutDataTypeStr=uint32
  Data Store Read : DataStoreRead  DataStoreName=RxID_CAN2
  Data Store Read1 : DataStoreRead  DataStoreName=fcn_call_counter
  Data Store Read10 : DataStoreRead  DataStoreName=Rx_State_CAN2
  Data Store Read4 : DataStoreRead  DataStoreName=Rx_State_CAN2
  Data Store Read9 : DataStoreRead  DataStoreName=Rx_State_CAN2
  Data Store Write : DataStoreWrite  DataStoreName=fcn_call_counter
  Equal{3,5..7} (4 alike) : RelationalOperator  Operator===  OutDataTypeStr=boolean  RndMeth=Simplest
  Equal4 : RelationalOperator  OutDataTypeStr=boolean  RndMeth=Simplest
  Prepare buffer : Subsystem  TreatAsAtomicUnit=on
  RxID_CAN : Subsystem
  Sum1 : Sum
  Update message buffers : Subsystem
  wires:
  Data Store Read4/1 -> Equal5/1
  Constant/1 -> Equal3/1
  Data Store Read10/1 -> Equal6/1
  Equal7/1 -> AND3/1
  AND2/1 -> Buffer ready/Enable
  Equal3/1 -> AND2/2
  Equal6/1 -> AND2/1
  Equal4/1 -> AND3/2
  Data Store Read9/1 -> Equal7/1
  Equal5/1 -> Prepare buffer/Enable
  Constant5/1 -> Equal7/2
  RxID_CAN/1(CAN_new) -> Equal4/1, Equal3/2
  Constant6/1 -> Equal5/2
  Constant7/1 -> Equal6/2
  RxID_CAN/2(message) -> Update message buffers/1(message)
  AND3/1 -> Update message buffers/Enable
  Data Store Read/1 -> RxID_CAN/1(RxID)  "RxID_CAN2_s"
  Sum1/1 -> Data Store Write/1  "RxCAN2_counter_s"
  Data Store Read1/1 -> Sum1/2
  Constant3/1 -> Sum1/1
  Constant4/1 -> Equal4/2

== system HANcoder_E407_TTA_Template_group2/HANcoder STM32 Target - E407-STM32 algorithm/TTA CAN System/CAN2 Send ==
  note: Logic Analyzer - DEBUG
      | Message in transmission!
  note: Function call counter
  note: DEBUG
  note: Logic Analyzer - DEBUG
  note: Transmission message count
      | Update
  note: Logic Analyzer - COMM Delay
  Trigger : TriggerPort  TriggerType=function-call  VariantControl=Variant  PortDimensions=1
  AND : Logic  IconShape=distinctive  AllPortsSameDT=off  OutDataTypeStr=boolean
  Bus Selector : BusSelector  OutputSignals=Buffer_1,Buffer_2,Buffer_3,Buffer_4,Buffer_5,Buffer_6,Buffer_7,Buffer_8
  CAN send1 : Subsystem  Tag=HANcoder_TARGET_STM32_E407  AncestorBlock=HANcoder_STM32_Target/STM32-E407/CAN/CAN/CAN send  mask(CAN send){canBus=CAN 2, frameType=Standard (11 bit), inputNumber=8, dataType=uint8, byteOrder=off, tsamp=-1}
      mask prompts: canBus "CAN channel"; frameType "Identifier type"; inputNumber "Input ports"; dataType "Input datatype"; byteOrder "Byte order: Checked = MSB first, unchecked = LSB first."; tsamp "Sample time"
      mask help:
      | Function
      | ==========
      | Send a message on the CAN channel.
      |
      | Parameters
      | ==========
      | CAN channel:           The CAN channel to send the message on.
      | Identifier type:         normal or extended ID's
      | Input ports:              The amount of input ports
      | Input datatype:        The datatype of the input ports
      | Byte order:               Select MSB or LSB first
      | Sample time:            -1 or divisible by base sample time [seconds]
      |
      | Input
      | ==========
      | Port 1:                   CAN ID(uint32) in hexadecimal ie: hex2dec('0a')
      | Port 2..9                CAN message data
      mask init:
      | sfcn_can_send_mcb(canBus, frameType, inputNumber, dataType, byteOrder)
      settings: MoveFcn=drawLogos
      mask Help: web('sfcn_can_send.html');
      mask TypeOptions canBus: CAN 1 | CAN 2
      mask TypeOptions frameType: Standard (11 bit) | Extended (29 bit)
      mask TypeOptions dataType: int8 | uint8 | int16 | uint16 | int32 | uint32 | boolean
      mask Display:
      | fprintf('Send on\nCAN %x', canBus);
      | port_label('input', 1, 'ID');patch([140 146 146],[8 14 2],[1 0 0]);patch([148 148 154],[14 2 8],[0 0 0.35]);
  Cast To Double : DataTypeConversion  OutDataTypeStr=double
  Constant : Constant  OutDataTypeStr=boolean
  Constant1 : Constant  Value=Sync_ID
  Constant2 : Constant  Value=LA_COMM_dly
  Constant3 : Constant  OutDataTypeStr=uint32
  Constant8 : Constant  Priority=2
  Data Store Memory1 : DataStoreMemory  DataStoreName=fcn_call_counter  ReadBeforeWriteMsg=warning  WriteAfterWriteMsg=warning  WriteAfterReadMsg=warning  ShowAdditionalParam=off  OutDataTypeStr=uint32
  Data Store Read : DataStoreRead  DataStoreName=fcn_call_counter
  Data Store Read1 : DataStoreRead  DataStoreName=TxID_CAN2
  Data Store Read2 : DataStoreRead  DataStoreName=Msg_Tx_CAN2
  Data Store Read3 : DataStoreRead  DataStoreName=TxID_CAN2
  Data Store Read4 : DataStoreRead  Priority=1  DataStoreName=Tx_msg_count_CAN2
  Data Store Write : DataStoreWrite  DataStoreName=fcn_call_counter
  Data Store Write1 : DataStoreWrite  DataStoreName=Toggle_Pin_A0
  Data Store Write2 : DataStoreWrite  Priority=4  DataStoreName=Tx_msg_count_CAN2
  Data Type Conversion{,4..10} (8 alike) : DataTypeConversion  OutDataTypeStr=uint8
  Data Type Conversion1 : DataTypeConversion  OutDataTypeStr=uint32
  Equal : RelationalOperator  Operator===  OutDataTypeStr=boolean  RndMeth=Simplest
  Logic Analyzer - COMM delay measurement : Subsystem  TreatAsAtomicUnit=on
  Plus : Sum  Priority=3
  Sum1 : Sum
  Terminator : Terminator
  wires:
  Constant/1 -> Data Store Write1/1
  Sum1/1 -> Data Store Write/1  "TxCAN2_counter_s"
  Data Store Read/1 -> Sum1/2
  Constant3/1 -> Sum1/1
  Data Type Conversion7/1 -> CAN send1/6(In6)
  Data Type Conversion6/1 -> CAN send1/5(In5)
  Data Type Conversion4/1 -> CAN send1/3(In3)
  Data Type Conversion5/1 -> CAN send1/4(In4)
  Data Type Conversion8/1 -> CAN send1/7(In7)
  Data Type Conversion9/1 -> CAN send1/8(In8)
  Data Type Conversion1/1 -> CAN send1/1(In1)
  Data Type Conversion/1 -> CAN send1/2(In2)
  Data Type Conversion10/1 -> CAN send1/9(In9)
  Data Store Read3/1 -> Data Type Conversion1/1  "TxID_CAN2_s"
  Bus Selector/3 -> Data Type Conversion5/1  "<Buffer_3>"
  Bus Selector/2 -> Data Type Conversion4/1  "<Buffer_2>"
  Bus Selector/6 -> Data Type Conversion8/1  "<Buffer_6>"
  Bus Selector/4 -> Data Type Conversion6/1  "<Buffer_4>"
  Bus Selector/8 -> Data Type Conversion10/1  "<Buffer_8>"
  Data Store Read2/1 -> Bus Selector/1
  Bus Selector/7 -> Data Type Conversion9/1  "<Buffer_7>"
  Bus Selector/5 -> Data Type Conversion7/1  "<Buffer_5>"
  Data Store Read4/1 -> Plus/1
  Plus/1 -> Data Store Write2/1
  Constant8/1 -> Plus/2
  Bus Selector/1 -> Cast To Double/1, Data Type Conversion/1  "<Buffer_1>"
  Cast To Double/1 -> Terminator/1  "Tx_temporal_msg_CAN2"
  Constant1/1 -> Equal/2
  Constant2/1 -> AND/2
  AND/1 -> Logic Analyzer - COMM delay measurement/Enable
  Equal/1 -> AND/1
  Data Store Read1/1 -> Equal/1

== system HANcoder_E407_TTA_Template_group2/HANcoder STM32 Target - E407-STM32 algorithm/TTA CAN System/If Action Subsystem ==
  note: CAN ID Init
  Action Port : ActionPort  ActionType=then
  Add : Sum  Inputs=++++
  Constant : Constant
  Constant1 : Constant  Value=2
  Constant2 : Constant  Value=4
  Constant3 : Constant  Value=8
  Digital Input4 : HANcoder_STM32_Target/STM32-E407/Digital Inputs/Digital Input  Tag=HANcoder_TARGET_STM32_E407  pinID=CON3 - D2 - 5V Tolerant  config=Pulldown  tsamp=-1
      settings: SourceProductName=HANcoder STM32 Target
  Digital Input5 : HANcoder_STM32_Target/STM32-E407/Digital Inputs/Digital Input  Tag=HANcoder_TARGET_STM32_E407  pinID=CON3 - D3 - 5V Tolerant  config=Pulldown  tsamp=-1
      settings: SourceProductName=HANcoder STM32 Target
  Digital Input6 : HANcoder_STM32_Target/STM32-E407/Digital Inputs/Digital Input  Tag=HANcoder_TARGET_STM32_E407  pinID=CON3 - D4 - 5V Tolerant  config=Pulldown  tsamp=-1
      settings: SourceProductName=HANcoder STM32 Target
  Digital Input7 : HANcoder_STM32_Target/STM32-E407/Digital Inputs/Digital Input  Tag=HANcoder_TARGET_STM32_E407  pinID=CON3 - D5 - 5V Tolerant  config=Pulldown  tsamp=-1
      settings: SourceProductName=HANcoder STM32 Target
  Multiply{,1..3} (4 alike) : Product
  Out1 : Outport
  wires:
  Constant1/1 -> Multiply1/1
  Add/1 -> Out1/1
  Constant3/1 -> Multiply3/1
  Constant2/1 -> Multiply2/1
  Multiply2/1 -> Add/3
  Digital Input7/1 -> Multiply3/2
  Digital Input5/1 -> Multiply1/2
  Multiply3/1 -> Add/4
  Multiply1/1 -> Add/2
  Digital Input6/1 -> Multiply2/2
  Multiply/1 -> Add/1
  Digital Input4/1 -> Multiply/2
  Constant/1 -> Multiply/1

== system HANcoder_E407_TTA_Template_group2/HANcoder STM32 Target - E407-STM32 algorithm/TTA CAN System/Initialize Clock Schedule ==
  Enable : EnablePort
  Constant : Constant  OutDataTypeStr=uint16
  Constant1 : Constant  Value=3  OutDataTypeStr=uint8
  Constant2 : Constant
  Data Store Write : DataStoreWrite  DataStoreName=init_clock
  Schedule Compare Event : HANcoder_STM32_Target/STM32-E407/Timer Outputs/Schedule Compare Event  Tag=HANcoder_TARGET_STM32_E407  pin=TIM4 - CON PD - 15 - 5V Tolerant  tsamp=-1
      settings: SourceProductName=HANcoder STM32 Target
  wires:
  Constant/1 -> Schedule Compare Event/1
  Constant1/1 -> Schedule Compare Event/2
  Constant2/1 -> Data Store Write/1

== system HANcoder_E407_TTA_Template_group2/HANcoder STM32 Target - E407-STM32 algorithm/TTA CAN System/Local Time generation ==
  note: Reschedule IRQ activation
  Clock_State : Inport
  function : TriggerPort  TriggerType=function-call  VariantControl=Variant
  Chart : Stateflow chart  TreatAsAtomicUnit=on
  Constant : Constant  Value=frequency_IRQ  OutDataTypeStr=uint16
  Constant1 : Constant  Value=3  OutDataTypeStr=uint8
  Constant2 : Constant  OutDataTypeStr=uint16
  Data Store Read : DataStoreRead  DataStoreName=Local_Ticks
  Data Store Read1 : DataStoreRead  DataStoreName=Local_Ticks
  Data Store Write : DataStoreWrite  DataStoreName=Local_Ticks
  Get Last Event Counter : HANcoder_STM32_Target/STM32-E407/Timer Outputs/Get Last Event Counter  Tag=HANcoder_TARGET_STM32_E407  pin=TIM4 - CON PD - 15 - 5V Tolerant  tsamp=-1
      settings: SourceProductName=HANcoder STM32 Target
  Schedule Compare Event1 : HANcoder_STM32_Target/STM32-E407/Timer Outputs/Schedule Compare Event  Tag=HANcoder_TARGET_STM32_E407  pin=TIM4 - CON PD - 15 - 5V Tolerant  tsamp=-1
      settings: SourceProductName=HANcoder STM32 Target
  Sum : Sum
  Sum1 : Sum
  Switch : Switch  Criteria=u2 > Threshold
  activate_CAN_management : Outport
  wires:
  Get Last Event Counter/1 -> Sum/1
  Constant/1 -> Sum/2
  Sum/1 -> Schedule Compare Event1/1
  Constant1/1 -> Schedule Compare Event1/2
  Data Store Read1/1 -> Switch/3
  Data Store Read/1 -> Sum1/1
  Constant2/1 -> Sum1/2
  Clock_State/1 -> Chart/1(Condition), Switch/2
  Switch/1 -> Data Store Write/1  "local_ticks_interrupt"
  Sum1/1 -> Switch/1
  Chart/1(Trigger_Signal()) -> activate_CAN_management/1

== system HANcoder_E407_TTA_Template_group2/HANcoder STM32 Target - E407-STM32 algorithm/TTA CAN System/Measure EXecution time ==
  note: Measured Execution Time
  Trigger : TriggerPort  TriggerType=function-call  VariantControl=Variant
  Constant1 : Constant  Priority=1  Value=LA_MEX_Flag
  DEBUG - Toggle digital pin A3 : Subsystem  Priority=3
  Data Store Memory4 : DataStoreMemory  DataStoreName=A3_Pin_State  ReadBeforeWriteMsg=warning  WriteAfterWriteMsg=warning  WriteAfterReadMsg=warning  ShowAdditionalParam=off  OutDataTypeStr=boolean
  wires:
  Constant1/1 -> DEBUG - Toggle digital pin A3/Enable

== system HANcoder_E407_TTA_Template_group2/HANcoder STM32 Target - E407-STM32 algorithm/TTA CAN System/Output Compare Init ==
  S-Function : S-Function  FunctionName=sfcn_timeout_init  SFunctionDeploymentMode=off  EnableBusSupport=off
  Term1 : Terminator
  wires:
  S-Function/1 -> Term1/1
